simulink subsystem "Condenser_2Pass"  (R2022b)
settings: Solver=VariableStepAuto  StartTime=0.0  StopTime=10.0  RelTol=1e-3
model mask{p_init=101.325, p_init_unit=kPa, p_init_conf=compiletime, IC_spec=Specific Enthalpy, h_init=265, h_init_unit=kJ/kg, h_init_conf=compiletime, x_init=x0, x_init_conf=compiletime, energy_spec=foundation.enum.energy_spec.enthalpy}
  mask prompts: p_init "Initial pressure"; IC_spec "Initial fluid energy specification"; h_init "Initial specific enthalpy"; x_init "Initial vapor quality"; energy_spec "Initial fluid energy specification"
undefined symbols (not defined in the file): a_fins, a_maflow, a_x_cond, a_x_httubes, d_cond, l_man, N_row, N_tube_pass, v_ma
libraries: fl_lib x3, SimscapeFluids_lib x2
settings Model: Creator=emcgarri  LastModifiedBy=esmithzb
settings SolverCC: MaxZcPerStep=1
settings ModelReferenceCC: EnableRefExpFcnMdlSchedulingChecks=on

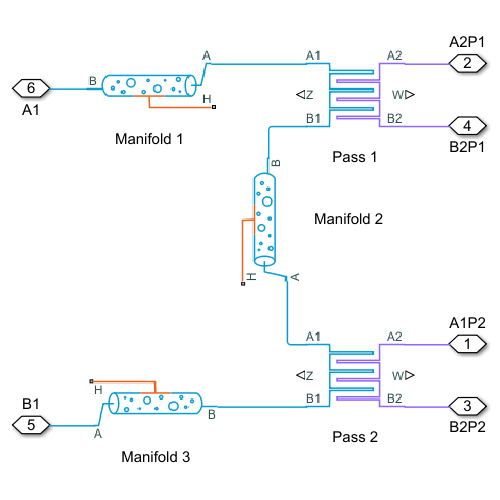
[thumbnail: Simulink's stored preview of the top-level diagram]
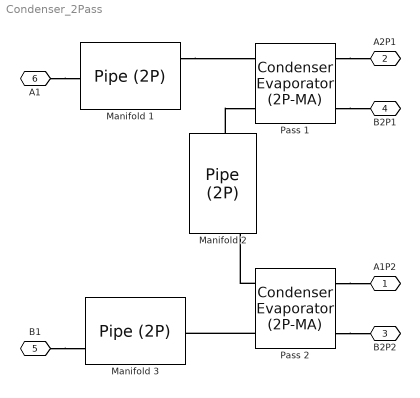
== system Condenser_2Pass ==
  Manifold 1 : fl_lib/Two-Phase Fluid/Elements/Pipe (2P)  length=l_man(1) cm  area=a_man cm^2  Dh=d_man cm  length_add=0 m  roughness=15e-6 m  Re_lam=2000  Re_tur=4000  shape_factor=64  Nu_lam=3.66  inertia=simscape.enum.onoff.off  energy_spec=energy_spec  p_init=p_init kPa  T_init=293.15 K  x_init=x0  alpha_init=0.5  h_init=h_init kJ/kg  u_init=1500 kJ/kg  mdot_init=0 kg/s  time_constant=0.1 s
      settings: InternalSimscapePortConfiguration="{\"Bottom\":[],\"Left\":[{\"id\":\"A\",\"label\":\"A\",\"type\":\"foundation.two_phase_fluid.two_phase_fluid\"},{\"id\":\"H\",\"label\":\"H\",\"type\":\"foundation.thermal.thermal\"}],\"Right\":[{\"id\":\"B\",\"label\":\"B\",\"type\":\"foundation.two_phase_fluid.two_phase_fluid\"}],\"Top\":[]}"
  Manifold 2 : fl_lib/Two-Phase Fluid/Elements/Pipe (2P)  length=l_man(2) cm  area=a_man cm^2  Dh=d_man cm  length_add=0 m  roughness=15e-6 m  Re_lam=2000  Re_tur=4000  shape_factor=64  Nu_lam=3.66  inertia=simscape.enum.onoff.off  energy_spec=energy_spec  p_init=p_init kPa  T_init=293.15 K  x_init=x0  alpha_init=0.5  h_init=h_init kJ/kg  u_init=1500 kJ/kg  mdot_init=0 kg/s  time_constant=0.1 s
      settings: InternalSimscapePortConfiguration="{\"Bottom\":[],\"Left\":[{\"id\":\"A\",\"label\":\"A\",\"type\":\"foundation.two_phase_fluid.two_phase_fluid\"},{\"id\":\"H\",\"label\":\"H\",\"type\":\"foundation.thermal.thermal\"}],\"Right\":[{\"id\":\"B\",\"label\":\"B\",\"type\":\"foundation.two_phase_fluid.two_phase_fluid\"}],\"Top\":[]}"
  Manifold 3 : fl_lib/Two-Phase Fluid/Elements/Pipe (2P)  length=l_man(3) cm  area=a_man cm^2  Dh=d_man cm  length_add=0 m  roughness=15e-6 m  Re_lam=2000  Re_tur=4000  shape_factor=64  Nu_lam=3.66  inertia=simscape.enum.onoff.off  energy_spec=energy_spec  p_init=p_init kPa  T_init=293.15 K  x_init=x0  alpha_init=0.5  h_init=h_init kJ/kg  u_init=1500 kJ/kg  mdot_init=0 kg/s  time_constant=0.1 s
      settings: InternalSimscapePortConfiguration="{\"Bottom\":[],\"Left\":[{\"id\":\"A\",\"label\":\"A\",\"type\":\"foundation.two_phase_fluid.two_phase_fluid\"},{\"id\":\"H\",\"label\":\"H\",\"type\":\"foundation.thermal.thermal\"}],\"Right\":[{\"id\":\"B\",\"label\":\"B\",\"type\":\"foundation.two_phase_fluid.two_phase_fluid\"}],\"Top\":[]}"
  Pass 1 : SimscapeFluids_lib/Fluid Network Interfaces/Heat Exchangers/Condenser Evaporator (2P-MA)  flow_arrangement=fluids.interfaces.heat_exchangers.enum.FlowArrangement2PMA.Cross  cross_flow_arrangement=fluids.interfaces.heat_exchangers.enum.CrossFlowArrangement2PMA.UnmixedUnmixed  R_wall=0 K/kW  area_A1=a_cond cm^2  area_B1=a_cond cm^2  area_A2=a_x_cond(1) cm^2  area_B2=a_x_cond(1) cm^2  tube_num_2P=N_tube_pass(1)  tube_length_2P=l_tube cm  tube_cross_section_2P=fluids.interfaces.heat_exchangers.enum.TubeCrossSection.Rectangular  tube_diameter_2P=d_cond/8 cm  tube_width_2P=w_tube mm  tube_height_2P=h_tube mm  tube_inner_diameter_2P=0.05 m  tube_outer_diameter_2P=0.1 m  tube_flow_area_2P=a_tube mm^2  tube_wetted_perimeter_2P=p_tube mm  tube_heat_perimeter_2P=p_tube mm  tube_pressure_loss_spec_2P=fluids.interfaces.heat_exchangers.enum.TubePressureLossSpec2P.Haaland  tube_loss_coeff_2P=10  tube_length_add_2P=0 m  tube_roughness_pressure_2P=15e-6 m  tube_Re_lam_pressure_2P=2000  tube_Re_tur_pressure_2P=4000  tube_shape_factor_generic_2P=64  tube_heat_coeff_spec_2P=fluids.interfaces.heat_exchangers.enum.TubeHeatCoeffSpec2P.GneilinskiCavalliniZecchin  tube_colburn_coeff_liq_2P=[.023, .8, .33]  tube_colburn_coeff_mix_2P=[.05, .8, .33]  tube_colburn_coeff_vap_2P=[.023, .8, .33]  tube_roughness_heat_2P=15e-6 m  tube_Re_lam_heat_2P=2000  tube_Re_tur_heat_2P=4000  tube_Nu_lam_generic_2P=3.66  fouling_factor_2P=0.1 K*m^2/kW  fin_area_2P=0 m^2  fin_efficiency_2P=0.5  energy_spec_2P=energy_spec  p_init_2P=p_init kPa  T_init_2P=293.15 K  x_init_2P=x0  alpha_init_2P=0.5  h_init_2P=h_init kJ/kg  u_init_2P=1500 kJ/kg  flow_geometry_MA=fluids.interfaces.heat_exchangers.enum.FlowGeometryMA.Generic  tube_num_MA=25  tube_length_MA=1 m  tube_cross_section_MA=fluids.interfaces.heat_exchangers.enum.TubeCrossSection.Circular  tube_diameter_MA=0.05 m  tube_width_MA=0.05 m  tube_height_MA=0.05 m  tube_inner_diameter_MA=0.05 m  tube_outer_diameter_MA=0.1 m  tube_flow_area_MA=0.002 m^2  tube_wetted_perimeter_MA=0.15 m  tube_heat_perimeter_MA=0.15 m  tube_pressure_loss_spec_MA=fluids.interfaces.heat_exchangers.enum.TubePressureLossSpec.Haaland  tube_loss_coeff_MA=10  tube_length_add_MA=0.1 m  tube_roughness_pressure_MA=15e-6 m  tube_Re_lam_pressure_MA=2000  tube_Re_tur_pressure_MA=4000  tube_shape_factor_generic_MA=64  tube_heat_coeff_spec_MA=fluids.interfaces.heat_exchangers.enum.TubeHeatCoeffSpec.Gneilinski  tube_colburn_coeff_MA=[.023, .8, .33]  tube_roughness_heat_MA=15e-6 m  tube_Re_lam_heat_MA=2000  tube_Re_tur_heat_MA=4000  tube_Nu_lam_generic_MA=3.66  bank_arrangement_MA=fluids.interfaces.heat_exchangers.enum.BankArrangement.Inline  bank_num_rows_MA=N_tube_row  bank_tubes_per_row_MA=N_row(1)  bank_width_MA=w_cond cm  bank_tube_diameter_MA=d_cond cm  bank_longitudinal_pitch_MA=1.5*d_cond cm  bank_transverse_pitch_MA=1.5*d_cond cm  bank_pressure_loss_spec_MA=fluids.interfaces.heat_exchangers.enum.BankPressureLossSpec.Martin  bank_euler_MA=10  bank_heat_coeff_spec_MA=fluids.interfaces.heat_exchangers.enum.BankHeatCoeffSpec.Martin  bank_colburn_coeff_MA=[.27, .63, .36]  generic_flow_area_MA=a_maflow(1) cm^2  generic_heat_area_MA=a_x_httubes(1) cm^2  generic_volume_MA=v_ma(1) cm^3  generic_loss_coeff_MA=10  generic_colburn_coeff_MA=REPRabc  fouling_factor_MA=0.1 K*m^2/kW  fin_area_MA=a_fins(1) m^2  fin_efficiency_MA=0.5  p_init_MA=0.101325 MPa  T_init_MA=T_air_cond degC  moisture_spec_MA=foundation.enum.moisture_spec.relative_humidity  RH_init_MA=0.5  x_w_init_MA=0.01  y_w_init_MA=0.01  HR_init_MA=0.01  trace_gas_spec_MA=foundation.enum.trace_gas_spec.mass_fraction  x_g_init_MA=0.001  y_g_init_MA=0.001  RH_ws_MA=1
      settings: InternalSimscapePortConfiguration="{\"Bottom\":[],\"Left\":[{\"id\":\"A1\",\"label\":\"A1\",\"type\":\"foundation.two_phase_fluid.two_phase_fluid\"},{\"id\":\"Z\",\"label\":\"Z\",\"type\":\"output\"},{\"id\":\"B1\",\"label\":\"B1\",\"type\":\"foundation.two_phase_fluid.two_phase_fluid\"}],\"Right\":[{\"id\":\"A2\",\"label\":\"A2\",\"type\":\"foundation.moist_air.moist_air\"},{\"id\":\"W\",\"label\":\"W\",\"type\":\"output\"},{\"id\":\"B2\",\"label\":\"B2\",\"type\":\"foundation.moist_air.moist_air\"}],\"Top\":[]}"
  Pass 2 : SimscapeFluids_lib/Fluid Network Interfaces/Heat Exchangers/Condenser Evaporator (2P-MA)  flow_arrangement=fluids.interfaces.heat_exchangers.enum.FlowArrangement2PMA.Cross  cross_flow_arrangement=fluids.interfaces.heat_exchangers.enum.CrossFlowArrangement2PMA.UnmixedUnmixed  R_wall=0 K/kW  area_A1=a_cond cm^2  area_B1=a_cond cm^2  area_A2=a_x_cond(2) cm^2  area_B2=a_x_cond(2) cm^2  tube_num_2P=N_tube_pass(2)  tube_length_2P=l_tube cm  tube_cross_section_2P=fluids.interfaces.heat_exchangers.enum.TubeCrossSection.Rectangular  tube_diameter_2P=d_cond/8 cm  tube_width_2P=w_tube mm  tube_height_2P=h_tube mm  tube_inner_diameter_2P=0.05 m  tube_outer_diameter_2P=0.1 m  tube_flow_area_2P=a_tube mm^2  tube_wetted_perimeter_2P=p_tube mm  tube_heat_perimeter_2P=p_tube mm  tube_pressure_loss_spec_2P=fluids.interfaces.heat_exchangers.enum.TubePressureLossSpec2P.Haaland  tube_loss_coeff_2P=10  tube_length_add_2P=0 m  tube_roughness_pressure_2P=15e-6 m  tube_Re_lam_pressure_2P=2000  tube_Re_tur_pressure_2P=4000  tube_shape_factor_generic_2P=64  tube_heat_coeff_spec_2P=fluids.interfaces.heat_exchangers.enum.TubeHeatCoeffSpec2P.GneilinskiCavalliniZecchin  tube_colburn_coeff_liq_2P=[.023, .8, .33]  tube_colburn_coeff_mix_2P=[.05, .8, .33]  tube_colburn_coeff_vap_2P=[.023, .8, .33]  tube_roughness_heat_2P=15e-6 m  tube_Re_lam_heat_2P=2000  tube_Re_tur_heat_2P=4000  tube_Nu_lam_generic_2P=3.66  fouling_factor_2P=0.1 K*m^2/kW  fin_area_2P=a_fins(2) m^2  fin_efficiency_2P=0.5  energy_spec_2P=energy_spec  p_init_2P=p_init kPa  T_init_2P=293.15 K  x_init_2P=x0  alpha_init_2P=0.5  h_init_2P=h_init kJ/kg  u_init_2P=1500 kJ/kg  flow_geometry_MA=fluids.interfaces.heat_exchangers.enum.FlowGeometryMA.Generic  tube_num_MA=25  tube_length_MA=1 m  tube_cross_section_MA=fluids.interfaces.heat_exchangers.enum.TubeCrossSection.Circular  tube_diameter_MA=0.05 m  tube_width_MA=0.05 m  tube_height_MA=0.05 m  tube_inner_diameter_MA=0.05 m  tube_outer_diameter_MA=0.1 m  tube_flow_area_MA=0.002 m^2  tube_wetted_perimeter_MA=0.15 m  tube_heat_perimeter_MA=0.15 m  tube_pressure_loss_spec_MA=fluids.interfaces.heat_exchangers.enum.TubePressureLossSpec.Haaland  tube_loss_coeff_MA=10  tube_length_add_MA=0.1 m  tube_roughness_pressure_MA=15e-6 m  tube_Re_lam_pressure_MA=2000  tube_Re_tur_pressure_MA=4000  tube_shape_factor_generic_MA=64  tube_heat_coeff_spec_MA=fluids.interfaces.heat_exchangers.enum.TubeHeatCoeffSpec.Gneilinski  tube_colburn_coeff_MA=[.023, .8, .33]  tube_roughness_heat_MA=15e-6 m  tube_Re_lam_heat_MA=2000  tube_Re_tur_heat_MA=4000  tube_Nu_lam_generic_MA=3.66  bank_arrangement_MA=fluids.interfaces.heat_exchangers.enum.BankArrangement.Inline  bank_num_rows_MA=N_tube_row  bank_tubes_per_row_MA=N_row(2)  bank_width_MA=w_cond cm  bank_tube_diameter_MA=d_cond cm  bank_longitudinal_pitch_MA=1.5*d_cond cm  bank_transverse_pitch_MA=1.5*d_cond cm  bank_pressure_loss_spec_MA=fluids.interfaces.heat_exchangers.enum.BankPressureLossSpec.Martin  bank_euler_MA=10  bank_heat_coeff_spec_MA=fluids.interfaces.heat_exchangers.enum.BankHeatCoeffSpec.Martin  bank_colburn_coeff_MA=[.27, .63, .36]  generic_flow_area_MA=a_maflow(2) cm^2  generic_heat_area_MA=a_x_httubes(2) cm^2  generic_volume_MA=v_ma(2) cm^3  generic_loss_coeff_MA=10  generic_colburn_coeff_MA=REPRabc  fouling_factor_MA=0.1 K*m^2/kW  fin_area_MA=a_fins(2) m^2  fin_efficiency_MA=0.5  p_init_MA=0.101325 MPa  T_init_MA=T_air_cond degC  moisture_spec_MA=foundation.enum.moisture_spec.relative_humidity  RH_init_MA=0.5  x_w_init_MA=0.01  y_w_init_MA=0.01  HR_init_MA=0.01  trace_gas_spec_MA=foundation.enum.trace_gas_spec.mass_fraction  x_g_init_MA=0.001  y_g_init_MA=0.001  RH_ws_MA=1
      settings: InternalSimscapePortConfiguration="{\"Bottom\":[],\"Left\":[{\"id\":\"A1\",\"label\":\"A1\",\"type\":\"foundation.two_phase_fluid.two_phase_fluid\"},{\"id\":\"Z\",\"label\":\"Z\",\"type\":\"output\"},{\"id\":\"B1\",\"label\":\"B1\",\"type\":\"foundation.two_phase_fluid.two_phase_fluid\"}],\"Right\":[{\"id\":\"A2\",\"label\":\"A2\",\"type\":\"foundation.moist_air.moist_air\"},{\"id\":\"W\",\"label\":\"W\",\"type\":\"output\"},{\"id\":\"B2\",\"label\":\"B2\",\"type\":\"foundation.moist_air.moist_air\"}],\"Top\":[]}"
  A1P2 : PMIOPort  Side=Right
  A2P1 : PMIOPort  Port=2  Side=Right
  B2P2 : PMIOPort  Port=3  Side=Right
  B2P1 : PMIOPort  Port=4  Side=Right
  B1 : PMIOPort  Port=5  Side=Left
  A1 : PMIOPort  Port=6  Side=Left
  connections:
  Pass 2/LConn3 -- Manifold 3/RConn1
  Manifold 2/RConn1 -- Pass 1/LConn3
  Pass 2/RConn1 -- A1P2/RConn1
  Pass 1/RConn3 -- B2P1/RConn1
  Pass 1/RConn1 -- A2P1/RConn1
  Pass 2/RConn3 -- B2P2/RConn1
  Manifold 1/LConn1 -- Pass 1/LConn1
  B1/RConn1 -- Manifold 3/LConn1
  A1/RConn1 -- Manifold 1/RConn1
  Pass 2/LConn1 -- Manifold 2/LConn1
